simulink model "exampleAVB"  (Simulink 7.8)
settings: Solver=ode45  StartTime=0.0  StopTime=inf  FixedStep=0.1  MaxStep=0.005  MinStep=0.005  RelTol=1e-12
libraries: model_lib x4
settings Model: Creator=mohammad  LastModifiedBy=mai03
settings DebuggingCC: SolverPrmCheckMsg=none  FcnCallInpInsideContextMsg=Use local settings  UnconnectedInputMsg=none  UnconnectedOutputMsg=none  UnconnectedLineMsg=none

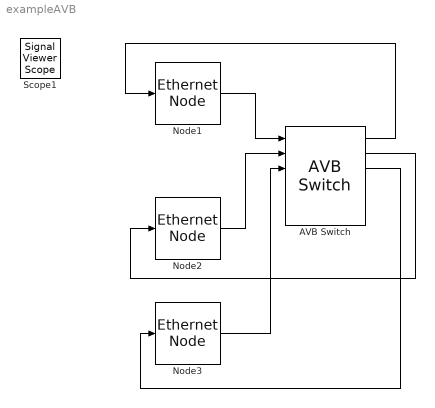
== system exampleAVB ==
  AVB Switch : model_lib/AVB Switch  Priority=1  avb_number=1
  Node1 : model_lib/Ethernet Node  node_number=1
  Node2 : model_lib/Ethernet Node  node_number=2
  Node3 : model_lib/Ethernet Node  node_number=3
  Scope1 : SignalViewerScope  IOType=viewer  RefreshTime=0.035000
  wires:
  Node1/1 -> AVB Switch/1
  AVB Switch/1 -> Node1/1
  Node2/1 -> AVB Switch/2
  Node3/1 -> AVB Switch/3
  AVB Switch/2 -> Node2/1
  AVB Switch/3 -> Node3/1
